simulink model "car_model"  (R2019b)
settings: Solver=ode23tb  StartTime=0.0  StopTime=30  RelTol=1e-3
InitFcn:
  | CommonVariables
  | Klqr5Velocities
values from neighbouring files (symbols this model uses):
  BattChrgMax = -80000    [CommonVariables.m]
  BattDischrgMax = 80000    [CommonVariables.m]
  BrkPrsMax = 5000000    [CommonVariables.m]
  ChrgLmt_bpt = [1 1 1 1 1 1 1 1 0.7 0.35 0]    [CommonVariables.m]
  DischrgLmt_bpt = [0 0.35 0.7 1 1 1 1 1 1 1 1]    [CommonVariables.m]
  disk_abore = 0.05    [CommonVariables.m]
  DLCXref = [0 7 9 18 33.5 34 42 50 60]    [CommonVariables.m]
  DLCYref = [0 0 -4.5 -4 -3.75 1.25 0.75 0 0]    [CommonVariables.m]
  efficiency_table = [85 85 85 85 85 85 85 85 85 85 85 85 85 85 85;85 85 85 85 85 85 85 85 85 85 85 85 85 85 85;85 85 90 90 90 90 90 90 90 90 88 88 88 88 88;85 85 92 92 92 92 92 92 92 92 92 90 90 90 90;85 85 92 92 93 93 93 93 92 92 92 90 90 90 90;85 85 93 94 94 94 94 94 94 94 94 94 94 94 94;85 85 93 94 94 95 95 95 95 95 95 95 95 95 95;85 85 93 94 94 95 95 95 95 95 95 95 95 95 95;85 85 93 94 95 95 95 95 95 95 95 95 95  ...(+141 chars)    [CommonVariables.m]
  F0z = [2886 2907]    [CommonVariables.m]
  h = 0.134    [CommonVariables.m]
  MotSpd = [0 1000 2000 2728.370453 3000 4000 5000 6000 7000 8000 9000 10000]    [CommonVariables.m]
  MotTrq = [280 280 280 280 254.6479089 190.9859317 152.7887454 127.3239545 109.1348181 95.49296586 84.88263632 76.39437268]    [CommonVariables.m]
  mu_kinetic = 0.35    [CommonVariables.m]
  Ndiff = 7.94    [CommonVariables.m]
  num_pads = 2    [CommonVariables.m]
  RegenBrkCutOff = [0 1]    [CommonVariables.m]
  RegenBrkSpd_bpt = [5 9]    [CommonVariables.m]
  Rm = 0.15    [CommonVariables.m]
  SOC_bpt = [0 10 20 30 40 50 60 70 80 90 100]    [CommonVariables.m]
  T_eff_bp = [0 20 40 60 80 100 120 140 160 180 200 220 240 260 280]    [CommonVariables.m]
  w_eff_bp = [0 1000 2000 2728.370453 3000 4000 5000 6000 7000 8000 9000 10000]    [CommonVariables.m]
undefined symbols (not defined in the file or in its folder): A_1, A_2, A_3, A_4, A_5, B1_1, B1_2, B1_3, B1_4, B1_5, Disabled, Discovery, Klqr1, Klqr2, Klqr3, Klqr4, Klqr5, Right, Serial, STM32F4, VEH
libraries: simulink x10, vehdynlibtire x8, vehdynlibsuspension x7, vehdynlibscenariocommon x5, autolibutils x4, sim3dlib x4, autolibmappedmotor x4, autolibshared x2, sharedtransform x2, vehdynlibviscommon x2, pil_lib x1, vehdynlibdriver x1
(part 3 of 7)

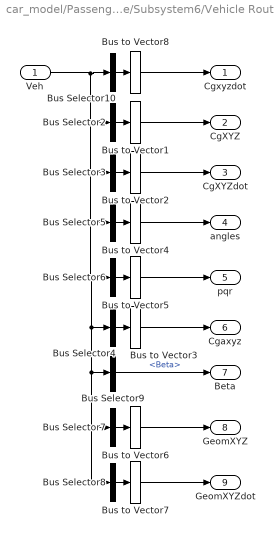
== system car_model/Passenger Vehicle/Subsystem6/Vehicle Routing ==
  Veh : Inport
  Bus Selector10 : BusSelector  OutputSignals=BdyFrm.Cg.Vel.xdot,BdyFrm.Cg.Vel.ydot,BdyFrm.Cg.Vel.zdot  OutputAsBus=on
  Bus Selector2 : BusSelector  OutputSignals=InertFrm.Cg.Disp.X,InertFrm.Cg.Disp.Y,InertFrm.Cg.Disp.Z  OutputAsBus=on
  Bus Selector3 : BusSelector  OutputSignals=InertFrm.Cg.Vel.Xdot,InertFrm.Cg.Vel.Ydot,InertFrm.Cg.Vel.Zdot  OutputAsBus=on
  Bus Selector4 : BusSelector  OutputSignals=BdyFrm.Cg.Acc.ax,BdyFrm.Cg.Acc.ay,BdyFrm.Cg.Acc.az  OutputAsBus=on
  Bus Selector5 : BusSelector  OutputSignals=InertFrm.Cg.Ang.phi,InertFrm.Cg.Ang.theta,InertFrm.Cg.Ang.psi  OutputAsBus=on
  Bus Selector6 : BusSelector  OutputSignals=BdyFrm.Cg.AngVel.p,BdyFrm.Cg.AngVel.q,BdyFrm.Cg.AngVel.r  OutputAsBus=on
  Bus Selector7 : BusSelector  OutputSignals=InertFrm.Geom.Disp.X,InertFrm.Geom.Disp.Y,InertFrm.Geom.Disp.Z  OutputAsBus=on
  Bus Selector8 : BusSelector  OutputSignals=InertFrm.Geom.Vel.Xdot,InertFrm.Geom.Vel.Ydot,InertFrm.Geom.Vel.Zdot  OutputAsBus=on
  Bus Selector9 : BusSelector  OutputSignals=BdyFrm.Geom.Ang.Beta
  Bus to Vector{1..8} (8 alike) : BusToVector
  Cgxyzdot : Outport  VectorParamsAs1DForOutWhenUnconnected=off
  CgXYZ : Outport  Port=2  VectorParamsAs1DForOutWhenUnconnected=off
  CgXYZdot : Outport  Port=3  VectorParamsAs1DForOutWhenUnconnected=off
  angles : Outport  Port=4  VectorParamsAs1DForOutWhenUnconnected=off
  pqr : Outport  Port=5  VectorParamsAs1DForOutWhenUnconnected=off
  Cgaxyz : Outport  Port=6  VectorParamsAs1DForOutWhenUnconnected=off
  Beta : Outport  Port=7  VectorParamsAs1DForOutWhenUnconnected=off
  GeomXYZ : Outport  Port=8  VectorParamsAs1DForOutWhenUnconnected=off
  GeomXYZdot : Outport  Port=9  VectorParamsAs1DForOutWhenUnconnected=off
  wires:
  Bus Selector3/1 -> Bus to Vector2/1
  Bus to Vector1/1 -> CgXYZ/1
  Bus to Vector5/1 -> pqr/1
  Bus Selector5/1 -> Bus to Vector4/1
  Bus Selector6/1 -> Bus to Vector5/1
  Bus to Vector4/1 -> angles/1
  Bus to Vector8/1 -> Cgxyzdot/1
  Bus Selector2/1 -> Bus to Vector1/1
  Bus Selector8/1 -> Bus to Vector7/1
  Bus to Vector6/1 -> GeomXYZ/1
  Bus Selector9/1 -> Beta/1  "<Beta>"
  Bus Selector4/1 -> Bus to Vector3/1
  Bus Selector10/1 -> Bus to Vector8/1
  Bus to Vector7/1 -> GeomXYZdot/1
  Bus to Vector3/1 -> Cgaxyz/1
  Bus Selector7/1 -> Bus to Vector6/1
  Bus to Vector2/1 -> CgXYZdot/1
  Veh/1 -> Bus Selector8/1, Bus Selector7/1, Bus Selector9/1, Bus Selector4/1, Bus Selector6/1, Bus Selector5/1, Bus Selector3/1, Bus Selector2/1, Bus Selector10/1

== system car_model/Passenger Vehicle/Subsystem6/Wheel Routing ==
  Info : Inport
  Wheel : Inport  Port=2
  Bus Selector : BusSelector  OutputSignals=InertFrm.FrntAxl.Lft.Disp.Y,InertFrm.FrntAxl.Rght.Disp.Y,InertFrm.RearAxl.Lft.Disp.Y,InertFrm.RearAxl.Rght.Disp.Y
  Bus Selector1 : BusSelector  OutputSignals=InertFrm.FrntAxl.Lft.Disp.X,InertFrm.FrntAxl.Rght.Disp.X,InertFrm.RearAxl.Lft.Disp.X,InertFrm.RearAxl.Rght.Disp.X
  Bus Selector2 : BusSelector  OutputSignals=TireFrame.z,TireFrame.omega,TireFrame.Kappa,TireFrame.Alpha
  Bus Selector3 : BusSelector  OutputSignals=InertFrm.FrntAxl.Lft.Disp.Z,InertFrm.FrntAxl.Rght.Disp.Z,InertFrm.RearAxl.Lft.Disp.Z,InertFrm.RearAxl.Rght.Disp.Z
  Bus Selector4 : BusSelector  OutputSignals=BdyFrm.FrntAxl.Lft.Disp.z,BdyFrm.FrntAxl.Rght.Disp.z,BdyFrm.RearAxl.Lft.Disp.z,BdyFrm.RearAxl.Rght.Disp.z
  Subtract : Sum  Inputs=-+-
  Vector Concatenate{1..4} (4 alike) : Concatenate  NumInputs=4
  XWheel : Outport  Unit=m  VectorParamsAs1DForOutWhenUnconnected=off
  YWheel : Outport  Port=2  Unit=m  VectorParamsAs1DForOutWhenUnconnected=off
  ZWheel : Outport  Port=3  PortDimensions=4  VectorParamsAs1DForOutWhenUnconnected=off
  omega : Outport  Port=4  PortDimensions=4  VectorParamsAs1DForOutWhenUnconnected=off
  kappa : Outport  Port=5  PortDimensions=4  VectorParamsAs1DForOutWhenUnconnected=off
  alpha : Outport  Port=6  PortDimensions=4  VectorParamsAs1DForOutWhenUnconnected=off
  wires:
  Bus Selector1/4 -> Vector Concatenate2/4  "<X>"
  Bus Selector/1 -> Vector Concatenate1/1  "<Y>"
  Bus Selector1/3 -> Vector Concatenate2/3  "<X>"
  Bus Selector/4 -> Vector Concatenate1/4  "<Y>"
  Bus Selector1/2 -> Vector Concatenate2/2  "<X>"
  Bus Selector/3 -> Vector Concatenate1/3  "<Y>"
  Bus Selector/2 -> Vector Concatenate1/2  "<Y>"
  Vector Concatenate1/1 -> YWheel/1
  Bus Selector1/1 -> Vector Concatenate2/1  "<X>"
  Vector Concatenate2/1 -> XWheel/1
  Bus Selector2/1 -> Subtract/3  "<z>"
  Bus Selector2/2 -> omega/1  "<omega>"
  Bus Selector2/3 -> kappa/1  "<Kappa>"
  Bus Selector2/4 -> alpha/1  "<Alpha>"
  Wheel/1 -> Bus Selector2/1
  Subtract/1 -> ZWheel/1
  Info/1 -> Bus Selector1/1, Bus Selector4/1, Bus Selector3/1, Bus Selector/1
  Bus Selector3/2 -> Vector Concatenate3/2  "<Z>"
  Bus Selector3/3 -> Vector Concatenate3/3  "<Z>"
  Bus Selector3/4 -> Vector Concatenate3/4  "<Z>"
  Bus Selector3/1 -> Vector Concatenate3/1  "<Z>"
  Vector Concatenate3/1 -> Subtract/2
  Vector Concatenate4/1 -> Subtract/1
  Bus Selector4/1 -> Vector Concatenate4/1  "<z>"
  Bus Selector4/4 -> Vector Concatenate4/4  "<z>"
  Bus Selector4/3 -> Vector Concatenate4/3  "<z>"
  Bus Selector4/2 -> Vector Concatenate4/2  "<z>"

== system car_model/Passenger Vehicle/Subsystem6/Wheels and Tires ==
  Suspension : Inport
  Axle Torque : Inport  Port=2
  Brake Press : Inport  Port=3  Unit=Pa
  Ground Input : Inport  Port=4
  Friction : Inport  Port=5  PortDimensions=4
  Bus Selector1 : BusSelector  OutputSignals=Whl.Ang,Whl.F,Whl.AngVel,Whl.xdot,Whl.ydot
  Constant3 : Constant  Value=zeros(4,1)
  Cont LPF : autolibutils/Cont LPF  wc=100*2*pi  aMode=2
      settings: SourceProductName=Powertrain Blockset  SourceProductBaseCode=PW
  Cont LPF1 : autolibutils/Cont LPF  wc=100*2*pi  aMode=2
      settings: SourceProductName=Powertrain Blockset  SourceProductBaseCode=PW
  Manual Switch6 : ManualSwitch
  Matrix Concatenate : Concatenate  NumInputs=3  Mode=Multidimensional array
  Reshape1 : Reshape
  Reshape2 : Reshape
  Saturation : Saturate  UpperLimit=inf  LowerLimit=-10*9.81*2000  ZeroCross=off
  Selector : Selector  NumberOfDimensions=2  InputPortWidth=3  IndexOptions=Index vector (dialog),Select all  Indices=[3],1  OutputSizes=1,1
  Selector1 : Selector  NumberOfDimensions=2  InputPortWidth=1  IndexOptions=Index vector (dialog),Select all  Indices=[3],1  OutputSizes=1,1
  Selector2 : Selector  NumberOfDimensions=2  InputPortWidth=3  IndexOptions=Index vector (dialog),Select all  Indices=3,1  OutputSizes=1,1
  Selector3 : Selector  NumberOfDimensions=2  InputPortWidth=3  IndexOptions=Index vector (dialog),Select all  Indices=1,1  OutputSizes=1,1
  Terminator{,1,3..5} (5 alike) : Terminator
  VDBS : Subsystem  VariantControl=0
  Wheels : Outport  VectorParamsAs1DForOutWhenUnconnected=off
  wires:
  VDBS/1(Wheels) -> Wheels/1  "Wheels"
  Bus Selector1/2 -> Selector/1  "<F>"
  VDBS/2(FrntAxlF) -> Terminator/1
  VDBS/3(RearAxlF) -> Terminator1/1
  VDBS/4(omega) -> Terminator3/1
  VDBS/5(SteerTrq) -> Terminator4/1
  Selector1/1 -> Reshape1/1
  Matrix Concatenate/1 -> VDBS/7(VehVel)
  Axle Torque/1 -> VDBS/3(AxleTrq)
  Selector2/1 -> VDBS/1(WheelAng)  "Wheel Angles"
  Constant3/1 -> Manual Switch6/1
  Manual Switch6/1 -> VDBS/2(CamberAng)  "Camber Angles"
  Selector/1 -> Reshape2/1
  Saturation/1 -> VDBS/5(Fz)
  Ground Input/1 -> VDBS/8(Ground Level)
  VDBS/7(SuspWhlVz) -> Matrix Concatenate/3  "zdot"
  Bus Selector1/1 -> Cont LPF1/1  "<Ang>"
  Selector3/1 -> Manual Switch6/2  "Camber Angles"
  Suspension/1 -> Bus Selector1/1
  Bus Selector1/4 -> Matrix Concatenate/1  "<xdot>"
  Bus Selector1/5 -> Matrix Concatenate/2  "<ydot>"
  VDBS/6(SuspWhlPz) -> Terminator5/1  "z"
  Reshape2/1 -> Cont LPF/1
  Bus Selector1/3 -> Selector1/1  "<AngVel>"
  Reshape1/1 -> VDBS/6(r)
  Brake Press/1 -> VDBS/4(BrkPrs)
  Friction/1 -> VDBS/9(Friction)
  Cont LPF/1 -> Saturation/1
  Cont LPF1/1 -> Selector3/1, Selector2/1

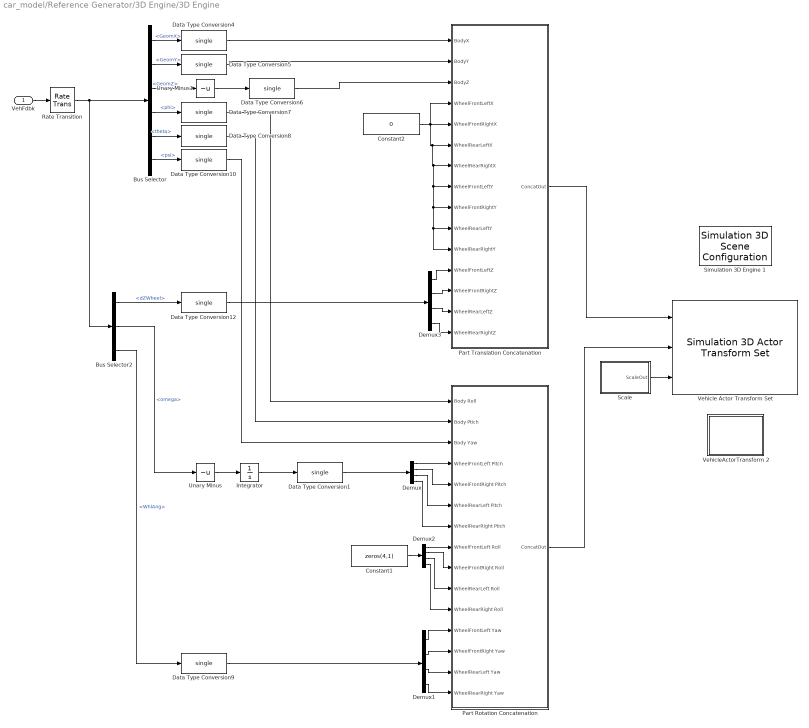
== system car_model/Reference Generator/3D Engine/3D Engine ==
  VehFdbk : Inport
  Bus Selector : BusSelector  OutputSignals=Body.GeomX,Body.GeomY,Body.GeomZ,Body.phi,Body.theta,Body.psi
  Bus Selector2 : BusSelector  OutputSignals=Wheels.dZWheel,Wheels.omega,Driveline.WhlAng
  Constant1 : Constant  Value=zeros(4,1)  OutDataTypeStr=single
  Constant2 : Constant  Value=0  OutDataTypeStr=single
  Data Type Conversion{1,4..10,12} (9 alike) : DataTypeConversion  OutDataTypeStr=single
  Demux{,1..3} (4 alike) : Demux
  Integrator : Integrator  WrapState=on  WrappedStateUpperValue=2*pi  WrappedStateLowerValue=0  ZeroCross=off
  Part Rotation Concatenation : Subsystem
  Part Translation Concatenation : Subsystem
  Rate Transition : RateTransition  OutPortSampleTime=dt3D
  Scale : Subsystem
  Simulation 3D Engine 1 : sim3dlib/Simulation 3D Scene Configuration  Priority=1  SceneDesc=Open surface  vehTagList={'Scene Origin'}  vehTag=Scene Origin  OpVisEn=off  Ts=dt3D  ProjectFormat=Executable  ProjectName=VehicleSimulation.exe  sensorTag=MainCamera1  sensorId=1  sensorName=MainCamera1  mountLoc=Origin  offsetFlag=off  tmountOffset=[0, 0, 0]  rmountOffset=[0, 0, 0]  HorizontalResolution=1280  VerticalResolution=720  HorizontalFOV=60  mountPoint=[0 0 0]  mountOrientation=[0 0 0]  aMode=aMode  ID=1
      settings: AttributesFormatString=Priority: %<Priority>  SourceProductName=Vehicle Dynamics Blockset  SourceProductBaseCode=VE
  Unary Minus : UnaryMinus
  Unary Minus1 : UnaryMinus
  Vehicle Actor Transform Set : sim3dlib/Simulation 3D Actor Transform Set  ActorTag=SimulinkVehicle1  NumberOfParts=5  CustNumOfParts=3  Translation=[X_o Y_o -Z_o; 0 0 0; 0 0 0; 0 0 0; 0 0 0]  Rotation=[phi_o theta_o psi_o; 0 0 0; 0 0 0; 0 0 0; 0 0 0]  Scale=[1 1 1; 1 1 1; 1 1 1; 1 1 1; 1 1 1]  Ts=dt3D  aMode=1
      settings: SourceProductName=Vehicle Dynamics Blockset  SourceProductBaseCode=VE
  VehicleActorTransform 2 : Subsystem  mask{depth=-5}
      mask prompts: depth "Initital Z position, depth (m):"
  wires:
  Unary Minus1/1 -> Data Type Conversion6/1
  Unary Minus/1 -> Integrator/1
  Bus Selector2/1 -> Data Type Conversion12/1  "<dZWheel>"
  Rate Transition/1 -> Bus Selector/1, Bus Selector2/1
  Scale/1(ScaleOut) -> Vehicle Actor Transform Set/3
  Demux/4 -> Part Rotation Concatenation/7(WheelRearRight Ptich)
  Demux/3 -> Part Rotation Concatenation/6(WheelRearLeft Pitch)
  Demux/2 -> Part Rotation Concatenation/5(WheelFrontRight Pitch)
  Demux/1 -> Part Rotation Concatenation/4(WheelFrontLeft Pitch)
  Constant1/1 -> Demux2/1
  Bus Selector/4 -> Data Type Conversion7/1  "<phi>"
  Part Rotation Concatenation/1(ConcatOut) -> Vehicle Actor Transform Set/2
  Part Translation Concatenation/1(ConcatOut) -> Vehicle Actor Transform Set/1
  Data Type Conversion12/1 -> Demux3/1
  Demux3/4 -> Part Translation Concatenation/15(WheelRearRightZ)
  Demux3/3 -> Part Translation Concatenation/14(WheelRearLeftZ)
  Demux3/1 -> Part Translation Concatenation/12(WheelFrontLeftZ)
  Demux3/2 -> Part Translation Concatenation/13(WheelFrontRightZ)
  VehFdbk/1 -> Rate Transition/1
  Data Type Conversion6/1 -> Part Translation Concatenation/3(BodyZ)
  Demux1/4 -> Part Rotation Concatenation/15(WheelRearRight Yaw)
  Demux1/3 -> Part Rotation Concatenation/14(WheelRearLeft Yaw)
  Demux2/1 -> Part Rotation Concatenation/8(WheelFrontLeft Roll)
  Demux2/2 -> Part Rotation Concatenation/9(WheelFrontRight Roll)
  Demux2/3 -> Part Rotation Concatenation/10(WheelRearLeft Roll)
  Demux2/4 -> Part Rotation Concatenation/11(WheelRearRight Roll)
  Bus Selector2/3 -> Data Type Conversion9/1  "<WhlAng>"
  Bus Selector2/2 -> Unary Minus/1  "<omega>"
  Data Type Conversion9/1 -> Demux1/1
  Demux1/1 -> Part Rotation Concatenation/12(WheelFrontLeft Yaw)
  Demux1/2 -> Part Rotation Concatenation/13(WheelFrontRight Yaw)
  Integrator/1 -> Data Type Conversion1/1
  Data Type Conversion1/1 -> Demux/1
  Data Type Conversion8/1 -> Part Rotation Concatenation/2(Body Ptich)
  Data Type Conversion5/1 -> Part Translation Concatenation/2(BodyY)
  Data Type Conversion10/1 -> Part Rotation Concatenation/3(Body Yaw)
  Constant2/1 -> Part Translation Concatenation/5(WheelFrontRightX), Part Translation Concatenation/6(WheelRearLeftX), Part Translation Concatenation/7(WheelRearRightX), Part Translation Concatenation/8(WheelFrontLeftY), Part Translation Concatenation/9(WheelFrontRightY), Part Translation Concatenation/10(WheelRearLeftY), Part Translation Concatenation/11(WheelRearRightY), Part Translation Concatenation/4(WheelFrontLeftX)
  Data Type Conversion4/1 -> Part Translation Concatenation/1(BodyX)
  Data Type Conversion7/1 -> Part Rotation Concatenation/1(Body Roll)
  Bus Selector/1 -> Data Type Conversion4/1  "<GeomX>"
  Bus Selector/2 -> Data Type Conversion5/1  "<GeomY>"
  Bus Selector/3 -> Unary Minus1/1  "<GeomZ>"
  Bus Selector/6 -> Data Type Conversion10/1  "<psi>"
  Bus Selector/5 -> Data Type Conversion8/1  "<theta>"

== system car_model/Reference Generator/3D Engine/3D Engine Disabled ==
  VehFdbk : Inport
  Terminator : Terminator
  wires:
  VehFdbk/1 -> Terminator/1

== system car_model/Reference Generator/Reference Generator/Constant Radius ==
  "VehFdbk " : Inport
  Bus Assignment : BusAssignment  AssignedSignals=Body.Y
  Bus Creator : BusCreator  Inputs=3
  Bus Creator1 : BusCreator  Inputs=4
  Bus Selector1 : BusSelector  OutputSignals=Body.ay
  Bus Selector2 : BusSelector  OutputSignals=Body.X,Body.Y,Body.psi,Body.Z
  Constant Radius : Subsystem  mask{Value=R, turnDirMask=Right}
      mask prompts: Value "Simulink:blkprm_prompts:ConstConstValue"; turnDirMask "Turn direction"
      mask TypeOptions Value: R/Value
      mask TypeOptions turnDirMask: Left | Right
      mask DialogControl Value Prompt: Constant value:
  Constant1 : Constant  Value=0
  Constant2 : Constant  Value=0
  Longitudinal Velocity Reference : Subsystem
  Signal Copy : SignalConversion  OverrideOpt=off
  ay Stop : vehdynlibscenariocommon/Slowly Increasing Steer/ay Stop  SystemSampleTime=-1  Latency=0  AutoFrameSizeCalculation=off
      settings: SourceProductName=Vehicle Dynamics Blockset  SourceProductBaseCode=VE
  " Vis" : Outport  VectorParamsAs1DForOutWhenUnconnected=off
  " Ref" : Outport  Port=2  VectorParamsAs1DForOutWhenUnconnected=off
  " Fdbk" : Outport  Port=3  VectorParamsAs1DForOutWhenUnconnected=off
  wires:
  Constant Radius/2(yFdbk) -> Bus Assignment/2
  Constant2/1 -> Bus Creator1/3  "Steer"
  Longitudinal Velocity Reference/1(xdot) -> Bus Creator1/1  "LngRef"
  Bus Creator1/1 -> " Ref"/1
  Constant1/1 -> Bus Creator1/4  "ThrotKill"
  Constant Radius/1(yRef) -> Bus Creator1/2  "LtrlRef"
  Bus Assignment/1 -> " Fdbk"/1
  Signal Copy/1 -> Bus Creator/3  "ZRef"
  Bus Creator/1 -> " Vis"/1
  Bus Selector2/4 -> Signal Copy/1  "<Z>"
  Constant Radius/4(YRef) -> Bus Creator/2  "YRef"
  "VehFdbk "/1 -> Bus Selector1/1, Bus Selector2/1, Bus Assignment/1
  Bus Selector2/2 -> Constant Radius/2(YVeh)  "<Y>"
  Bus Selector2/3 -> Constant Radius/3(psiVeh)  "<psi>"
  Bus Selector2/1 -> Constant Radius/1(XVeh)  "<X>"
  Constant Radius/3(XRef) -> Bus Creator/1  "XRef"
  Bus Selector1/1 -> ay Stop/1  "<ay>"

== system car_model/Reference Generator/Reference Generator/Double Lane Change ==
  "VehFdbk " : Inport
  Double Lane Change : vehdynlibscenariocommon/Lane Change Reference Generator  VariantControl=Variant1  t_start=t_start  XGate=XGate  xdot_r=xdot_r  xdotUnit=mph  xStart=xStart  vehW=vehW  lattoff=lattoff  centerSwitch=on  latRefbp=latRefbp  latRef=latRef  aMode=2
      settings: SourceProductName=Vehicle Dynamics Blockset  SourceProductBaseCode=VE
  " Vis" : Outport  VectorParamsAs1DForOutWhenUnconnected=off
  " Ref" : Outport  Port=2  VectorParamsAs1DForOutWhenUnconnected=off
  " Fdbk" : Outport  Port=3  VectorParamsAs1DForOutWhenUnconnected=off
  wires:
  Double Lane Change/2 -> " Ref"/1
  Double Lane Change/1 -> " Vis"/1
  "VehFdbk "/1 -> Double Lane Change/1, " Fdbk"/1

== system car_model/Reference Generator/Reference Generator/Increasing Steer ==
  "VehFdbk " : Inport
  Bus Creator : BusCreator  Inputs=3
  Ground : Ground
  Ground1 : Ground
  Ground2 : Ground
  Increasing Steer : vehdynlibscenariocommon/Slowly Increasing Steer  VariantControl=1  t_start=t_start  xdot_r=xdot_r  xdotUnit=mph  omega_hw=omega_hw  theta_max=theta_max  t_stop=t_stop  ay_max=ay_max  ay_stop=on  aMode=2
      settings: SourceProductName=Vehicle Dynamics Blockset  SourceProductBaseCode=VE
  " Vis" : Outport  VectorParamsAs1DForOutWhenUnconnected=off
  " Ref" : Outport  Port=2  VectorParamsAs1DForOutWhenUnconnected=off
  " Fdbk" : Outport  Port=3  VectorParamsAs1DForOutWhenUnconnected=off
  wires:
  Ground/1 -> Bus Creator/1  "XRef"
  Ground1/1 -> Bus Creator/2  "YRef"
  Ground2/1 -> Bus Creator/3  "ZRef"
  Increasing Steer/1 -> " Ref"/1  "LtrlRef"
  Bus Creator/1 -> " Vis"/1
  "VehFdbk "/1 -> Increasing Steer/1, " Fdbk"/1

== system car_model/Reference Generator/Reference Generator/Sine with Dwell ==
  "VehFdbk " : Inport
  Bus Creator : BusCreator  Inputs=3
  Ground : Ground
  Ground1 : Ground
  Ground2 : Ground
  Sine With Dwell : vehdynlibscenariocommon/Sine With Dwell  VariantControl=3  t_start=t_start  xdot_r=xdot_r  xdotUnit=mph  steerF=steerF  steerA=steerA  tdwell=tdwell  steerDir=off  aMode=2
      settings: SourceProductName=Vehicle Dynamics Blockset  SourceProductBaseCode=VE
  " Vis" : Outport  VectorParamsAs1DForOutWhenUnconnected=off
  " Ref" : Outport  Port=2  VectorParamsAs1DForOutWhenUnconnected=off
  " Fdbk" : Outport  Port=3  VectorParamsAs1DForOutWhenUnconnected=off
  wires:
  Ground/1 -> Bus Creator/1  "XRef"
  Ground1/1 -> Bus Creator/2  "YRef"
  Ground2/1 -> Bus Creator/3  "ZRef"
  Bus Creator/1 -> " Vis"/1
  "VehFdbk "/1 -> Sine With Dwell/1, " Fdbk"/1
  Sine With Dwell/1 -> " Ref"/1

== system car_model/Reference Generator/Reference Generator/Swept Sine ==
  "VehFdbk " : Inport
  Bus Creator : BusCreator  Inputs=3
  Ground : Ground
  Ground1 : Ground
  Ground2 : Ground
  Swept Sine : vehdynlibscenariocommon/Swept Sine Reference Generator  VariantControl=2  t_start=t_start  xdot_r=xdot_r  xdotUnit=mph  theta_hw=theta_hw  theta_hw_final=theta_hw_final  t_sweep=t_sweep  aMode=2
      settings: SourceProductName=Vehicle Dynamics Blockset  SourceProductBaseCode=VE
  " Vis" : Outport  VectorParamsAs1DForOutWhenUnconnected=off
  " Ref" : Outport  Port=2  VectorParamsAs1DForOutWhenUnconnected=off
  " Fdbk" : Outport  Port=3  VectorParamsAs1DForOutWhenUnconnected=off
  wires:
  Ground/1 -> Bus Creator/1  "XRef"
  Ground1/1 -> Bus Creator/2  "YRef"
  Ground2/1 -> Bus Creator/3  "ZRef"
  Bus Creator/1 -> " Vis"/1
  Swept Sine/1 -> " Ref"/1
  "VehFdbk "/1 -> Swept Sine/1, " Fdbk"/1

== system car_model/Visualization/ISO 15037-1:2006/Disabled ==
  VehFdbk : Inport
  Cntrl : Inport  Port=2
  Terminator : Terminator
  Terminator1 : Terminator
  wires:
  Cntrl/1 -> Terminator/1
  VehFdbk/1 -> Terminator1/1

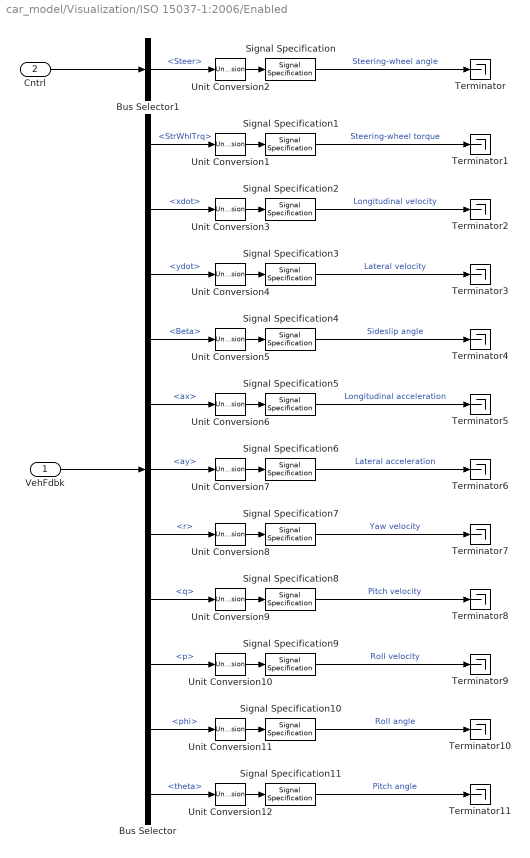
== system car_model/Visualization/ISO 15037-1:2006/Enabled ==
  VehFdbk : Inport
  Cntrl : Inport  Port=2
  Bus Selector : BusSelector  OutputSignals=Steering.StrWhlTrq,Body.xdot,Body.ydot,Body.Beta,Body.ax,Body.ay,Body.r,Body.q,Body.p,Body.phi,Body.theta
  Bus Selector1 : BusSelector  OutputSignals=Steer
  Signal Specification{,4,10..11} (4 alike) : SignalSpecification  Unit=deg
  Signal Specification1 : SignalSpecification  Unit=N*m
  Signal Specification2 : SignalSpecification  Unit=km/h
  Signal Specification3 : SignalSpecification  Unit=m/s
  Signal Specification5 : SignalSpecification  Unit=m/s^2
  Signal Specification6 : SignalSpecification  Unit=m/s^2
  Signal Specification7 : SignalSpecification  Unit=deg/s
  Signal Specification8 : SignalSpecification  Unit=deg/s
  Signal Specification9 : SignalSpecification  Unit=deg/s
  Terminator{,1..11} (12 alike) : Terminator
  Unit Conversion{1..12} (12 alike) : UnitConversion
  wires:
  Bus Selector/11 -> Unit Conversion12/1  "<theta>"
  Signal Specification11/1 -> Terminator11/1  "Pitch angle"
  Unit Conversion12/1 -> Signal Specification11/1
  Bus Selector/10 -> Unit Conversion11/1  "<phi>"
  Unit Conversion11/1 -> Signal Specification10/1
  Signal Specification10/1 -> Terminator10/1  "Roll angle"
  Bus Selector/9 -> Unit Conversion10/1  "<p>"
  Signal Specification9/1 -> Terminator9/1  "Roll velocity"
  Unit Conversion10/1 -> Signal Specification9/1
  Bus Selector/8 -> Unit Conversion9/1  "<q>"
  Unit Conversion9/1 -> Signal Specification8/1
  Signal Specification8/1 -> Terminator8/1  "Pitch velocity"
  Bus Selector/7 -> Unit Conversion8/1  "<r>"
  Signal Specification7/1 -> Terminator7/1  "Yaw velocity"
  Unit Conversion8/1 -> Signal Specification7/1
  Bus Selector/6 -> Unit Conversion7/1  "<ay>"
  Unit Conversion7/1 -> Signal Specification6/1
  Signal Specification6/1 -> Terminator6/1  "Lateral acceleration"
  Bus Selector/5 -> Unit Conversion6/1  "<ax>"
  Signal Specification5/1 -> Terminator5/1  "Longitudinal acceleration"
  Unit Conversion6/1 -> Signal Specification5/1
  Bus Selector/4 -> Unit Conversion5/1  "<Beta>"
  Unit Conversion5/1 -> Signal Specification4/1
  Signal Specification4/1 -> Terminator4/1  "Sideslip angle"
  Bus Selector/3 -> Unit Conversion4/1  "<ydot>"
  Signal Specification3/1 -> Terminator3/1  "Lateral velocity"
  Unit Conversion4/1 -> Signal Specification3/1
  Bus Selector/2 -> Unit Conversion3/1  "<xdot>"
  Unit Conversion3/1 -> Signal Specification2/1
  Signal Specification2/1 -> Terminator2/1  "Longitudinal velocity"
  Signal Specification1/1 -> Terminator1/1  "Steering-wheel torque"
  Unit Conversion1/1 -> Signal Specification1/1
  Bus Selector/1 -> Unit Conversion1/1  "<StrWhlTrq>"
  Signal Specification/1 -> Terminator/1  "Steering-wheel angle"
  Unit Conversion2/1 -> Signal Specification/1
  Bus Selector1/1 -> Unit Conversion2/1  "<Steer>"
  Cntrl/1 -> Bus Selector1/1
  VehFdbk/1 -> Bus Selector/1

== system car_model/Visualization/Scope Type/DLC ==
  VehFdbk : Inport
  Vis : Inport  Port=2
  Bus Creator : BusCreator  Inputs=3
  Bus Selector3 : BusSelector  OutputSignals=Body.Y,Body.X,Body.Z
  Bus Selector4 : BusSelector  OutputSignals=UB,LB,LtrlRef
  Lane Change : Scope
  Mux1 : Mux
  Signal Copy : SignalConversion  OverrideOpt=off
  Signal Copy1 : SignalConversion  OverrideOpt=off
  Signal Copy2 : SignalConversion  OverrideOpt=off
  Ref : Outport  VectorParamsAs1DForOutWhenUnconnected=off
  wires:
  Bus Selector4/1 -> Mux1/1  "<UB>"
  Bus Selector3/1 -> Mux1/4  "<Y>"
  VehFdbk/1 -> Bus Selector3/1
  Mux1/1 -> Lane Change/1
  Vis/1 -> Bus Selector4/1
  Bus Selector4/3 -> Signal Copy/1, Mux1/3  "<LtrlRef>"
  Bus Selector4/2 -> Mux1/2  "<LB>"
  Bus Selector3/2 -> Signal Copy1/1  "<X>"
  Bus Creator/1 -> Ref/1
  Bus Selector3/3 -> Signal Copy2/1  "<Z>"
  Signal Copy/1 -> Bus Creator/2  "YRef"
  Signal Copy1/1 -> Bus Creator/1  "XRef"
  Signal Copy2/1 -> Bus Creator/3  "ZRef"

== system car_model/Visualization/Scope Type/None ==
  VehFdbk : Inport
  Vis : Inport  Port=2
  Cntrl : Inport  Port=3
  Bus Selector1 : BusSelector  OutputSignals=Steer
  Bus Selector9 : BusSelector  OutputSignals=Body.r
  Signal Specification3 : SignalSpecification  Unit=deg/s
  Unit Conversion4 : UnitConversion
  Yaw Rate and Steer : Scope  NumInputPorts=2
  Ref : Outport  VectorParamsAs1DForOutWhenUnconnected=off
  wires:
  Bus Selector9/1 -> Unit Conversion4/1  "<r>"
  Signal Specification3/1 -> Yaw Rate and Steer/1
  Unit Conversion4/1 -> Signal Specification3/1
  VehFdbk/1 -> Bus Selector9/1  "VehFdbk"
  Bus Selector1/1 -> Yaw Rate and Steer/2  "<Steer>"
  Vis/1 -> Ref/1
  Cntrl/1 -> Bus Selector1/1

== system car_model/Visualization/Scope Type/XYZ ==
  VehFdbk : Inport
  Vis : Inport  Port=2
  Terminator : Terminator
  Ref : Outport  VectorParamsAs1DForOutWhenUnconnected=off
  wires:
  Vis/1 -> Ref/1
  VehFdbk/1 -> Terminator/1

== system car_model/Visualization/Vehicle XY Plotter/XY View ==
  VehFdbk : Inport
  Bus Selector1 : BusSelector  OutputSignals=Body.phi,Body.theta,Body.psi  OutputAsBus=on
  Bus Selector5 : BusSelector  OutputSignals=Driveline.WhlAng  OutputAsBus=on
  Bus Selector6 : BusSelector  OutputSignals=Body.GeomX,Body.GeomY,Body.GeomZ  OutputAsBus=on
  Bus Selector7 : BusSelector  OutputSignals=Body.GeomXdot,Body.GeomYdot,Body.GeomZdot  OutputAsBus=on
  Bus to Vector : BusToVector
  Bus to Vector1 : BusToVector
  Bus to Vector2 : BusToVector
  Vehicle XY Plotter : Subsystem  mask(Vehicle XY Plotter){a=VEH.FrontAxlePositionfromCG, b=VEH.RearAxlePositionfromCG, w=VEH.TrackWidth, figBorder=10, bufferSize=1024, extRef=off, pltDT=.1}
      mask prompts: a "Distance to front axle from CG, a [m]:"; b "Distance to rear axle from CG, b [m]:"; w "Track width, w [m]:"; figBorder "Distance to figure borders, figBorder [m]:"; bufferSize "Path buffer sampe size, bufferSize []:"; extRef "Plot path reference, extRef"; pltDT "Plot update rate, pltDT [s]:"
      mask help:
      | This block will display a MATLAB figure which indicates the vehicle path, current position and heading velocity.
      | An optional path reference is also provided.
      mask init:
      | if autoblkschecksimstopped(gcb)
      |     PortName = 'RefXYZ';
      |     InportOption  = {'built-in/Ground', [PortName, ' Ground'];...
      |         'built-in/Inport',PortName };
      |     if ~strcmp(get_param(gcb,'extRef'),'on')
      |         NewBlkHdl = autoblksreplaceblock(gcb, InportOption, 1);
      |         set_param(NewBlkHdl, 'ShowName', 'off');
      |     else
      |         autoblksreplaceblock(gcb, InportOption, 2);
      |     end
      | end
      mask TypeOptions a: Vehicle XY Plotter/a
      mask TypeOptions b: Vehicle XY Plotter/b
      mask TypeOptions w: Vehicle XY Plotter/w
      mask TypeOptions figBorder: Vehicle XY Plotter/figBorder
      mask TypeOptions bufferSize: Vehicle XY Plotter/bufferSize
  wires:
  Bus to Vector2/1 -> Vehicle XY Plotter/2(InertAng)
  Bus to Vector/1 -> Vehicle XY Plotter/1(InertXYZ)
  Bus Selector5/1 -> Vehicle XY Plotter/4(delta)
  Bus Selector1/1 -> Bus to Vector2/1
  Bus Selector6/1 -> Bus to Vector/1
  Bus Selector7/1 -> Bus to Vector1/1
  VehFdbk/1 -> Bus Selector6/1, Bus Selector1/1, Bus Selector7/1, Bus Selector5/1
  Bus to Vector1/1 -> Vehicle XY Plotter/3(InertXdotYdotZdot)

== system car_model/Visualization/Vehicle XY Plotter/XY View Ref ==
  VehFdbk : Inport
  Ref : Inport  Port=2
  Bus Selector1 : BusSelector  OutputSignals=Body.phi,Body.theta,Body.psi  OutputAsBus=on
  Bus Selector5 : BusSelector  OutputSignals=Driveline.WhlAng  OutputAsBus=on
  Bus Selector6 : BusSelector  OutputSignals=Body.GeomX,Body.GeomY,Body.GeomZ  OutputAsBus=on
  Bus Selector7 : BusSelector  OutputSignals=Body.GeomXdot,Body.GeomYdot,Body.GeomZdot  OutputAsBus=on
  Bus Selector8 : BusSelector  OutputSignals=XRef,YRef,ZRef  OutputAsBus=on
  Bus to Vector{,1..3} (4 alike) : BusToVector
  Vehicle XY Plotter : Subsystem  mask(Vehicle XY Plotter){a=VEH.FrontAxlePositionfromCG, b=VEH.RearAxlePositionfromCG, w=VEH.TrackWidth, figBorder=10, bufferSize=1024, extRef=on, pltDT=.1}
      mask prompts: a "Distance to front axle from CG, a [m]:"; b "Distance to rear axle from CG, b [m]:"; w "Track width, w [m]:"; figBorder "Distance to figure borders, figBorder [m]:"; bufferSize "Path buffer sampe size, bufferSize []:"; extRef "Plot path reference, extRef"; pltDT "Plot update rate, pltDT [s]:"
      mask help:
      | This block will display a MATLAB figure which indicates the vehicle path, current position and heading velocity.
      | An optional path reference is also provided.
      mask init: same as car_model/Visualization/Vehicle XY Plotter/XY View/Vehicle XY Plotter
      mask TypeOptions a: Vehicle XY Plotter/a
      mask TypeOptions b: Vehicle XY Plotter/b
      mask TypeOptions w: Vehicle XY Plotter/w
      mask TypeOptions figBorder: Vehicle XY Plotter/figBorder
      mask TypeOptions bufferSize: Vehicle XY Plotter/bufferSize
  wires:
  Bus Selector8/1 -> Bus to Vector3/1
  Bus to Vector1/1 -> Vehicle XY Plotter/3(InertXdotYdotZdot)
  VehFdbk/1 -> Bus Selector5/1, Bus Selector7/1, Bus Selector1/1, Bus Selector6/1
  Bus Selector7/1 -> Bus to Vector1/1
  Bus Selector6/1 -> Bus to Vector/1
  Bus Selector1/1 -> Bus to Vector2/1
  Bus Selector5/1 -> Vehicle XY Plotter/4(delta)
  Bus to Vector/1 -> Vehicle XY Plotter/1(InertXYZ)
  Bus to Vector2/1 -> Vehicle XY Plotter/2(InertAng)
  Ref/1 -> Bus Selector8/1
  Bus to Vector3/1 -> Vehicle XY Plotter/5(RefXYZ)

== system car_model/Controllers/Motor Torque Arbitration and Power Management/Power Management/Check Within Limits ==
  up : Inport
  u : Inport  Port=2
  lo : Inport  Port=3
  Compare To Zero : simulink/Logic and Bit Operations/Compare To Zero  relop=>=  OutDataTypeStr=boolean
  Compare To Zero1 : simulink/Logic and Bit Operations/Compare To Zero  relop=<=  OutDataTypeStr=boolean
  Logical Operator : Logic  AllPortsSameDT=off  OutDataTypeStr=boolean
  Saturation Dynamic1 : simulink/Discontinuities/Saturation Dynamic  OutMin=[]  OutMax=[]  OutDataTypeStr=Inherit: Same as second input  OutDataType=fixdt(1, 16)  OutScaling=2^-10  DoSatur=off
  Subtract : Sum  Inputs=+-
  Subtract1 : Sum  Inputs=-+
  InLimit : Outport  VectorParamsAs1DForOutWhenUnconnected=off
  y : Outport  Port=2  VectorParamsAs1DForOutWhenUnconnected=off
  wires:
  Saturation Dynamic1/1 -> y/1
  lo/1 -> Subtract1/2, Saturation Dynamic1/3
  up/1 -> Subtract/1, Saturation Dynamic1/1
  u/1 -> Subtract1/1, Subtract/2, Saturation Dynamic1/2
  Subtract/1 -> Compare To Zero/1
  Subtract1/1 -> Compare To Zero1/1
  Compare To Zero/1 -> Logical Operator/1
  Compare To Zero1/1 -> Logical Operator/2
  Logical Operator/1 -> InLimit/1

== system car_model/Controllers/Motor Torque Arbitration and Power Management/Power Management/Mech to Elec Power Estimate ==
  note: Check if Motoring
      | or Generating
  note: Using an Efficiency Map, we can estimate the
      | Electric Power from the Mechanical  Torque Request.
  note: Pelec_req = Pmech_req*Eff^k,
      | k = -1 if Motoring >= 0,
      | k = 1 if Generating < 0
  MotTrqCmd : Inport
  MotSpd : Inport  Port=2
  Abs : Abs
  Abs1 : Abs
  Constant1 : Constant  Value=-1  SampleTime=-1
  Constant2 : Constant  SampleTime=-1
  Eff Map : Lookup_n-D  BreakpointsForDimension1=w_eff_bp  BreakpointsForDimension2=T_eff_bp  Table=efficiency_table  ExtrapMethod=Clip  UseLastTableValue=on  InternalRulePriority=Speed  OutDataTypeStr=Inherit: Inherit from 'Table data'  RndMeth=Simplest  InputSameDT=on
  Gain1 : Gain  Gain=1/100
  Math Function : Math  Operator=pow  OutputSignalType=real  SaturateOnIntegerOverflow=on
  Product : Product
  Product3 : Product
  Product4 : Product
  Switch2 : Switch
  rads_to_rpm : Gain  Gain=30/pi
  MotPwrElecReq : Outport  VectorParamsAs1DForOutWhenUnconnected=off
  Eff2k : Outport  Port=2  VectorParamsAs1DForOutWhenUnconnected=off
  wires:
  Product3/1 -> Product4/1
  Switch2/1 -> Math Function/2
  Constant1/1 -> Switch2/1
  Constant2/1 -> Switch2/3
  Eff Map/1 -> Gain1/1
  Abs/1 -> Eff Map/1
  Gain1/1 -> Math Function/1
  Math Function/1 -> Eff2k/1, Product4/2
  Product4/1 -> MotPwrElecReq/1
  Abs1/1 -> Eff Map/2
  rads_to_rpm/1 -> Abs/1
  Product/1 -> Switch2/2
  MotSpd/1 -> Product3/1, Product/1, rads_to_rpm/1
  MotTrqCmd/1 -> Product3/2, Product/2, Abs1/1

== system car_model/Controllers/Motor Torque Arbitration and Power Management/Power Management/Torque Limit ==
  MotTrq : Inport
  MotSpd : Inport  Port=2
  Gain : Gain  Gain=-1
  MaxMotTrqVsSpd : Lookup_n-D  NumberOfTableDimensions=1  BreakpointsForDimension1=MotSpd  Table=MotTrq  ExtrapMethod=Clip  UseLastTableValue=on  InternalRulePriority=Speed  OutDataTypeStr=Inherit: Inherit from 'Table data'  RndMeth=Simplest  InputSameDT=on
  Saturation Dynamic : simulink/Discontinuities/Saturation Dynamic  OutMin=[]  OutMax=[]  OutDataTypeStr=Inherit: Same as second input  OutDataType=fixdt(1, 16)  OutScaling=2^-10  DoSatur=off
  rads_to_rpm : Gain  Gain=30/pi
  MotTrqCmd : Outport  VectorParamsAs1DForOutWhenUnconnected=off
  wires:
  MotTrq/1 -> Saturation Dynamic/2
  Saturation Dynamic/1 -> MotTrqCmd/1
  MotSpd/1 -> rads_to_rpm/1
  MaxMotTrqVsSpd/1 -> Gain/1, Saturation Dynamic/1
  rads_to_rpm/1 -> MaxMotTrqVsSpd/1
  Gain/1 -> Saturation Dynamic/3

== system car_model/Passenger Vehicle/Subsystem6/Suspension/Double Wishbone Suspension ==
  Wheel : Inport
  Steering : Inport  Port=2
  Vehicle : Inport  Port=3
  Bus Creator1 : BusCreator  Inputs=5
  Bus Creator2 : BusCreator  Inputs=2
  Bus Creator3 : BusCreator  Inputs=2
  Bus Creator4 : BusCreator  Inputs=6
  Bus Selector : BusSelector  OutputSignals=z,Re,zdot,Fx,Fy,M
  Bus Selector1 : BusSelector  OutputSignals=P,V
  Independent Suspension – Double Wishbone : vehdynlibsuspension/Independent Suspension - Double Wishbone  ActiveDampEn=off  NumAxl=2  NumTracksByAxl=[2 2]  StrgEnByAxl=[1 0]  AntiSwayEnByAxl=[1 0]  TrackNumVec="[1  2  1  2]"  AxleNumVec="[1  1  2  2]"  SuspTypesByAxle="[1  1]"  SuspImage=suspdw.png  IdealSuspEn=on  IdealSuspAxles="[1  2]"  Kz=Kz  F0z=F0z  Cz=Cz  Hmax=Hmax  f_act_susp_cz=[10000 10000;10000 10000]  f_act_susp_duty_bpt=[0 1]  f_act_susp_zdot_bpt=[-1 1]  Toe=0.  RollStrgSlp=0.  ToeStrgSlp=0.  Caster=0.  CasterHslp=0.  CasterStrgSlp=0.  Camber=0.  CamberHslp=0.  CamberStrgSlp=0.  StrgHgtSlp=0.1432  MappedSuspEn=off  MappedSuspAxles="[1  2]"  f_susp_axl_bp=[1 2]  f_susp_dz_bp=[-0.15 -0.14 -0.13 -0.12 -0.11 -0.10 -0.09 -0.08 -0.07 -0.06 -0.05 -0.04 -0.03 -0.02 -0.01 0.00 0.01 0.02 0.03 0.04 0.05 0.06 0.07 0.08 0.09 0.10 0.11 0.12 0.13 0.14 0.15]  f_susp_dzdot_bp=[-0.15 -0.14 -0.13 -0.12 -0.11 -0.10 -0.09 -0.08 -0.07 -0.06 -0.05 -0.04 -0.03 -0.02 -0.01 0.00 0.01 0.02 0.03 0.04 0.05 0.06 0.07 0.08 0.09 0.10 0.11 0.12 0.13 0.14 0.15]  f_susp_fmz=zeros(31,31,61,2,4)  f_susp_geom=zeros(31,61,2,3)  f_susp_strgdelta_bp=[-30,-29,-28,-27,-26,-25,-24,-23,-22,-21,-20,-19,-18,-17,-16,-15,-14,-13,-12,-11,-10,-9,-8,-7,-6,-5,-4,-3,-2,-1,0,1,2,3,4,5,6,7,8,9,10,11,12,13,14,15,16,17,18,19,20,21,22,23,24,25,26,27,28,29,30]  AntiSwayR=0.2  AntiSwayNtrlAng=0.5236  AntiSwayTrsK=8e2
      settings: SourceProductName=Vehicle Dynamics Blockset  SourceProductBaseCode=VE
  Selector1 : Selector  NumberOfDimensions=2  IndexOptions=Index vector (dialog),Select all  Indices=1,1  OutputSizes=1,1
  Selector2 : Selector  NumberOfDimensions=2  IndexOptions=Index vector (dialog),Select all  Indices=2,1  OutputSizes=1,1
  Steer Rate Adapter : Subsystem
  Steering Adapter : Subsystem
  Terminator : Terminator
  Vehicle Adapter : Subsystem
  Wheel  Adapter : Subsystem
  Suspension : Outport  VectorParamsAs1DForOutWhenUnconnected=off
  wires:
  Bus Creator3/1 -> Suspension/1
  Steering Adapter/1(StrgAng) -> Independent Suspension – Double Wishbone/9
  Independent Suspension – Double Wishbone/1 -> Terminator/1  "Susp"
  Wheel  Adapter/6(Re) -> Bus Creator4/6
  Bus Selector1/1 -> Independent Suspension – Double Wishbone/7  "<P>"
  Wheel  Adapter/2(WhlFy) -> Bus Creator4/2  "Fy"
  Wheel/1 -> Wheel  Adapter/1(Wheels)
  Steer Rate Adapter/1(AngVel) -> Bus Creator1/5  "AngVel"
  Bus Creator4/1 -> Bus Selector/1
  Bus Creator2/1 -> Bus Creator3/1  "Veh"
  Independent Suspension – Double Wishbone/5 -> Selector2/1, Selector1/1  "V"
  Selector2/1 -> Bus Creator1/3  "ydot"
  Bus Selector1/2 -> Independent Suspension – Double Wishbone/8  "<V>"
  Independent Suspension – Double Wishbone/2 -> Bus Creator2/1  "F"
  Bus Selector/2 -> Independent Suspension – Double Wishbone/2  "<Re>"
  Wheel  Adapter/5(M) -> Bus Creator4/5  "M"
  Bus Selector/4 -> Independent Suspension – Double Wishbone/4  "<Fx>"
  Independent Suspension – Double Wishbone/4 -> Bus Creator1/1  "F"
  Steering/1 -> Steering Adapter/1(Steer)
  Selector1/1 -> Bus Creator1/2  "xdot"
  Independent Suspension – Double Wishbone/3 -> Bus Creator2/2  "M"
  Vehicle Adapter/1(VehSusp) -> Bus Selector1/1
  Wheel  Adapter/4(zdot) -> Bus Creator4/4
  Vehicle/1 -> Steer Rate Adapter/1(Veh), Vehicle Adapter/1(Veh)
  Bus Selector/6 -> Independent Suspension – Double Wishbone/6  "<M>"
  Bus Selector/5 -> Independent Suspension – Double Wishbone/5  "<Fy>"
  Bus Selector/1 -> Independent Suspension – Double Wishbone/1  "<z>"
  Wheel  Adapter/3(z) -> Bus Creator4/3
  Independent Suspension – Double Wishbone/6 -> Bus Creator1/4  "Ang"
  Bus Creator1/1 -> Bus Creator3/2  "Whl"
  Wheel  Adapter/1(WhlFx) -> Bus Creator4/1  "Fx"
  Bus Selector/3 -> Independent Suspension – Double Wishbone/3  "<zdot>"

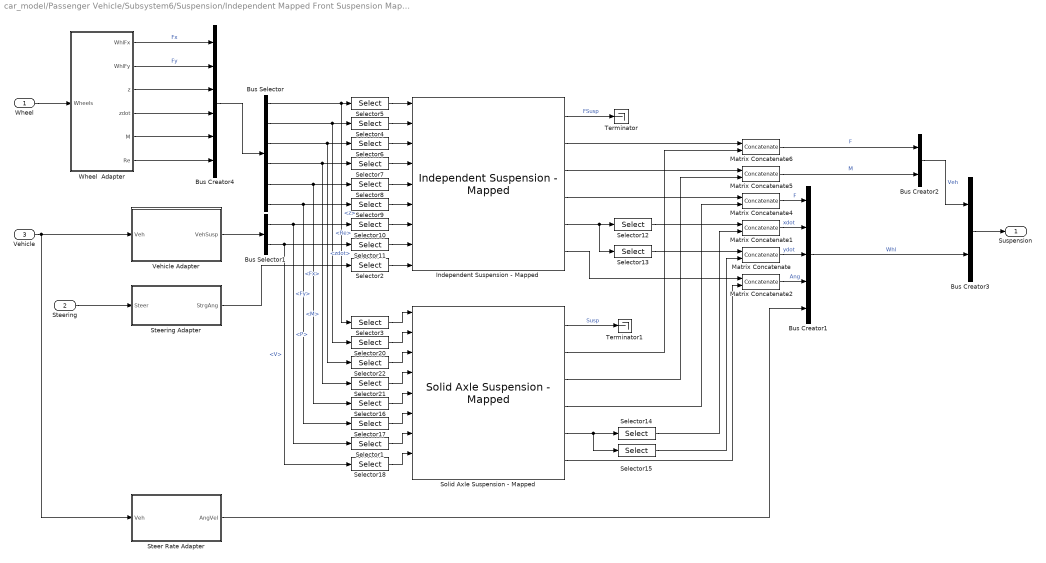
== system car_model/Passenger Vehicle/Subsystem6/Suspension/Independent Mapped Front Suspension Mapped Solid Axle Rear Suspension ==
  Wheel : Inport
  Steering : Inport  Port=2
  Vehicle : Inport  Port=3
  Bus Creator1 : BusCreator  Inputs=5
  Bus Creator2 : BusCreator  Inputs=2
  Bus Creator3 : BusCreator  Inputs=2
  Bus Creator4 : BusCreator  Inputs=6
  Bus Selector : BusSelector  OutputSignals=z,Re,zdot,Fx,Fy,M
  Bus Selector1 : BusSelector  OutputSignals=P,V
  Independent Suspension - Mapped : vehdynlibsuspension/Independent Suspension - Mapped  NumAxl=1  NumTracksByAxl=2  StrgEnByAxl=1  AntiSwayEnByAxl=1  TrackNumVec="[1  2]"  AxleNumVec="[1  1]"  SuspTypesByAxle=[2]  SuspImage=suspindmap.png  IdealSuspEn=off  IdealSuspAxles="[1  2]"  Kz=64370  F0z=9810  Cz=10000  Hmax=0.5  Toe=2  RollStrgSlp=-13  ToeStrgSlp=0.01  Caster=4  CasterHslp=-13  CasterStrgSlp=0.01  Camber=4  CamberHslp=-13  CamberStrgSlp=0.01  StrgHgtSlp=0.0025  MappedSuspEn=on  MappedSuspAxles=[1]  f_susp_axl_bp=[1 2]  f_susp_dz_bp=f_susp_dz_bp  f_susp_dzdot_bp=f_susp_dzdot_bp  f_susp_fmz=f_susp_fmz  f_susp_geom=f_susp_geom  f_susp_strgdelta_bp=f_susp_strgdelta_bp  NDFLookupOutType=1:4  NDGLookupOutType=1:3  AntiSwayR=0.2  AntiSwayNtrlAng=0.5236  AntiSwayTrsK=8e2
      link override For each track and axle combination calculate suspension forces and moments/Suspension/Suspension Angle Calculations: OverrideUsingVariant=MappedSteeringEnabled
      link override For each track and axle combination calculate suspension forces and moments/Suspension/Z axis suspension characteristic: OverrideUsingVariant=MappedSuspension
      settings: SourceProductName=Vehicle Dynamics Blockset  SourceProductBaseCode=VE
  Matrix Concatenate{,1..2,4..6} (6 alike) : Concatenate  Mode=Multidimensional array  ConcatenateDimension=2
  Selector1 : Selector  NumberOfDimensions=2  IndexOptions=Select all,Index vector (dialog)  Indices=[1 2],[3 4]  OutputSizes=1,1
  Selector10 : Selector  NumberOfDimensions=2  IndexOptions=Select all,Index vector (dialog)  Indices=[1 2],[1 2]  OutputSizes=1,1
  Selector11 : Selector  NumberOfDimensions=2  IndexOptions=Select all,Index vector (dialog)  Indices=[1 2],[1 2]  OutputSizes=1,1
  Selector12 : Selector  NumberOfDimensions=2  InputPortWidth=3  IndexOptions=Index vector (dialog),Select all  Indices=1,1  OutputSizes=1,1
  Selector13 : Selector  NumberOfDimensions=2  InputPortWidth=3  IndexOptions=Index vector (dialog),Select all  Indices=2,1  OutputSizes=1,1
  Selector14 : Selector  NumberOfDimensions=2  InputPortWidth=3  IndexOptions=Index vector (dialog),Select all  Indices=1,1  OutputSizes=1,1
  Selector15 : Selector  NumberOfDimensions=2  InputPortWidth=3  IndexOptions=Index vector (dialog),Select all  Indices=2,1  OutputSizes=1,1
  Selector{3,16,20..22} (5 alike) : Selector  IndexOptions=Index vector (dialog)  Indices=[3 4]  OutputSizes=1
  Selector17 : Selector  NumberOfDimensions=2  IndexOptions=Select all,Index vector (dialog)  Indices=[1 2],[3 4]  OutputSizes=1,1
  Selector18 : Selector  NumberOfDimensions=2  IndexOptions=Select all,Index vector (dialog)  Indices=[1 2],[3 4]  OutputSizes=1,1
  Selector{2,4..8} (6 alike) : Selector  IndexOptions=Index vector (dialog)  Indices=[1 2]  OutputSizes=1
  Selector9 : Selector  NumberOfDimensions=2  IndexOptions=Select all,Index vector (dialog)  Indices=[1 2],[1 2]  OutputSizes=1,1
  Solid Axle Suspension - Mapped : vehdynlibsuspension/Solid Axle Suspension - Mapped  NumAxl=1  NumTracksByAxl=2  StrgEnByAxl=0  TrackNumVec="[1  2]"  AxleNumVec="[1  1]"  SuspTypesByAxle=[2]  SuspImage=suspsamap.png  AxlIxx=AxlIxx  AxlM=AxlM  TrackCoords=[0 0;VEH.TrackWidth*[-1 1]/2;0 0]  SuspCoords=[0 0;VEH.TrackWidth*[-1 1]/2;0 0]  KzWhlAxl=KzWhlAxl  F0zWhlAxl=F0zWhlAxl  CzWhlAxl=CzWhlAxl  IdealSuspEn=off  IdealSuspAxles="[1  2]"  Kz=64370  F0z=9810  Cz=10000  Hmax=0.5  Toe=2  RollStrgSlp=-13  ToeStrgSlp=0.01  Caster=4  CasterHslp=-13  CasterStrgSlp=0.01  Camber=4  CamberHslp=-13  CamberStrgSlp=0.01  StrgHgtSlp=0.0025  MappedSuspEn=on  MappedSuspAxles=[1]  f_susp_axl_bp=[1 2]  f_susp_dz_bp=f_susp_dz_bp  f_susp_dzdot_bp=f_susp_dzdot_bp  f_susp_fmz=f_susp_fmz  f_susp_geom=f_susp_geom  f_susp_strgdelta_bp=f_susp_strgdelta_bp  NDFLookupOutType=1:4  NDGLookupOutType=1:3
      link override For each track and axle combination calculate suspension forces and moments/Suspension/Suspension Angle Calculations: OverrideUsingVariant=MappedSteeringEnabled
      link override For each track and axle combination calculate suspension forces and moments/Suspension/Z axis suspension characteristic: OverrideUsingVariant=MappedSuspension
      settings: SourceProductName=Vehicle Dynamics Blockset  SourceProductBaseCode=VE
  Steer Rate Adapter : Subsystem
  Steering Adapter : Subsystem
  Terminator : Terminator
  Terminator1 : Terminator
  Vehicle Adapter : Subsystem
  Wheel  Adapter : Subsystem
  Suspension : Outport  VectorParamsAs1DForOutWhenUnconnected=off
  wires:
  Solid Axle Suspension - Mapped/5 -> Selector15/1, Selector14/1
  Selector22/1 -> Solid Axle Suspension - Mapped/3
  Bus Selector/3 -> Selector22/1, Selector6/1  "<zdot>"
  Solid Axle Suspension - Mapped/4 -> Matrix Concatenate4/2
  Solid Axle Suspension - Mapped/1 -> Terminator1/1  "Susp"
  Selector12/1 -> Matrix Concatenate1/1
  Selector7/1 -> Independent Suspension - Mapped/4
  Selector18/1 -> Solid Axle Suspension - Mapped/8
  Selector13/1 -> Matrix Concatenate/1
  Selector14/1 -> Matrix Concatenate1/2
  Selector21/1 -> Solid Axle Suspension - Mapped/4
  Vehicle/1 -> Steer Rate Adapter/1(Veh), Vehicle Adapter/1(Veh)
  Wheel  Adapter/4(zdot) -> Bus Creator4/4
  Solid Axle Suspension - Mapped/3 -> Matrix Concatenate5/2
  Selector1/1 -> Solid Axle Suspension - Mapped/7
  Matrix Concatenate4/1 -> Bus Creator1/1  "F"
  Selector16/1 -> Solid Axle Suspension - Mapped/5
  Matrix Concatenate5/1 -> Bus Creator2/2  "M"
  Independent Suspension - Mapped/4 -> Matrix Concatenate4/1
  Selector4/1 -> Independent Suspension - Mapped/2
  Selector10/1 -> Independent Suspension - Mapped/7
  Selector9/1 -> Independent Suspension - Mapped/6
  Wheel  Adapter/3(z) -> Bus Creator4/3
  Solid Axle Suspension - Mapped/2 -> Matrix Concatenate6/2
  Wheel/1 -> Wheel  Adapter/1(Wheels)
  Selector5/1 -> Independent Suspension - Mapped/1
  Independent Suspension - Mapped/3 -> Matrix Concatenate5/1
  Selector8/1 -> Independent Suspension - Mapped/5
  Independent Suspension - Mapped/2 -> Matrix Concatenate6/1
  Independent Suspension - Mapped/6 -> Matrix Concatenate2/1
  Selector20/1 -> Solid Axle Suspension - Mapped/2
  Independent Suspension - Mapped/1 -> Terminator/1  "FSusp"
  Bus Creator2/1 -> Bus Creator3/1  "Veh"
  Bus Selector/4 -> Selector7/1, Selector21/1  "<Fx>"
  Independent Suspension - Mapped/5 -> Selector12/1, Selector13/1
  Matrix Concatenate2/1 -> Bus Creator1/4  "Ang"
  Wheel  Adapter/2(WhlFy) -> Bus Creator4/2  "Fy"
  Bus Creator4/1 -> Bus Selector/1
  Selector17/1 -> Solid Axle Suspension - Mapped/6
  Selector2/1 -> Independent Suspension - Mapped/9
  Wheel  Adapter/5(M) -> Bus Creator4/5
  Matrix Concatenate/1 -> Bus Creator1/3  "ydot"
  Steering/1 -> Steering Adapter/1(Steer)
  Matrix Concatenate1/1 -> Bus Creator1/2  "xdot"
  Selector15/1 -> Matrix Concatenate/2
  Selector3/1 -> Solid Axle Suspension - Mapped/1
  Bus Selector1/2 -> Selector11/1, Selector18/1  "<V>"
  Vehicle Adapter/1(VehSusp) -> Bus Selector1/1
  Steering Adapter/1(StrgAng) -> Selector2/1
  Selector6/1 -> Independent Suspension - Mapped/3
  Bus Selector/6 -> Selector9/1, Selector17/1  "<M>"
  Wheel  Adapter/1(WhlFx) -> Bus Creator4/1  "Fx"
  Selector11/1 -> Independent Suspension - Mapped/8
  Wheel  Adapter/6(Re) -> Bus Creator4/6
  Matrix Concatenate6/1 -> Bus Creator2/1  "F"
  Bus Selector1/1 -> Selector10/1, Selector1/1  "<P>"
  Solid Axle Suspension - Mapped/6 -> Matrix Concatenate2/2
  Bus Selector/1 -> Selector3/1, Selector5/1  "<z>"
  Bus Selector/5 -> Selector8/1, Selector16/1  "<Fy>"
  Bus Creator1/1 -> Bus Creator3/2  "Whl"
  Bus Creator3/1 -> Suspension/1
  Bus Selector/2 -> Selector20/1, Selector4/1  "<Re>"
  Steer Rate Adapter/1(AngVel) -> Bus Creator1/5
